simulink model "elevator"  (R2024b)
settings: Solver=VariableStepAuto  StartTime=0.0  StopTime=inf  RelTol=1e-3
settings Model: Creator=Admin  LastModifiedBy=Admin

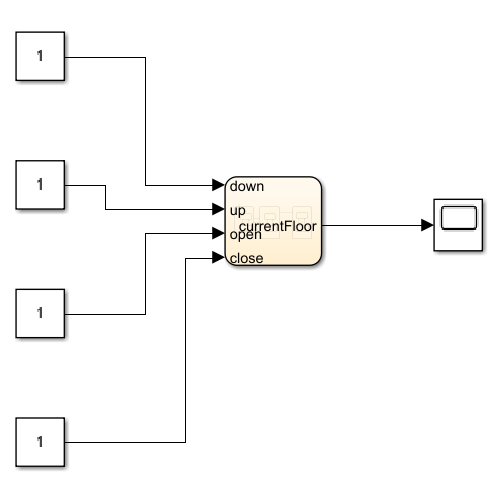
[thumbnail: Simulink's stored preview of the top-level diagram]
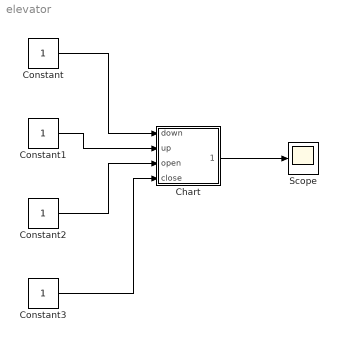
== system elevator ==
  Chart : Stateflow chart  TreatAsAtomicUnit=on
  Constant{,1..3} (4 alike) : Constant
  Scope : Scope
  wires:
  Chart/1(currentFloor) -> Scope/1
  Constant/1 -> Chart/1(down)
  Constant1/1 -> Chart/2(up)
  Constant2/1 -> Chart/3(open)
  Constant3/1 -> Chart/4(close)

== stateflow chart elevator/Chart ==
  state Floor1
    entry:
    currentFloor = 1;
    disp("Elevator on Floor 1");
    state Dooropen
      entry:
      disp("Door is open");
    state Doorclosed
      entry:
      disp("Door is closed");
    Floor1.Dooropen -> Floor1.Doorclosed : [close==1]
    Floor1.Doorclosed -> Floor1.Dooropen : [open==1]
  state Floor2
    entry:
    currentFloor = 2;
    disp("Elevator on Floor 2");
    state Dooropen
      entry:
      disp("Door is open");
    state Doorclosed
      entry:
      disp("Door is closed");
    Floor2.Dooropen -> Floor2.Doorclosed : [close==1]
    Floor2.Doorclosed -> Floor2.Dooropen : [open==1]
  state Floor3_
    entry:
    currentFloor = 3;
    disp("Elevator on Floor 3");
    state Dooropen
      entry:
      disp("Door is open");
    state Doorclosed_
      entry:
      disp("Door is closed");
    Floor3_.Dooropen -> Doorclosed_ : [close==1]
    Doorclosed_ -> Floor3_.Dooropen : [open==1]
  (default) -> Floor1
  Floor2 -> Floor3_ [order 1] : [up==1]
  Floor1 -> Floor2 : [up==1]
  Floor2 -> Floor1 [order 2] : [down==1]
  Floor3_ -> Floor2 : [down==1]
  data: down input; up input; currentFloor output; open input; close input
